simulink model "CNC_3_b"  (R2022b)
settings: Solver=VariableStepAuto  StartTime=0.0  StopTime=0.08  RelTol=1e-3
settings Model: Creator=Mahadevu Sudheer  LastModifiedBy=Mahadevu Sudheer

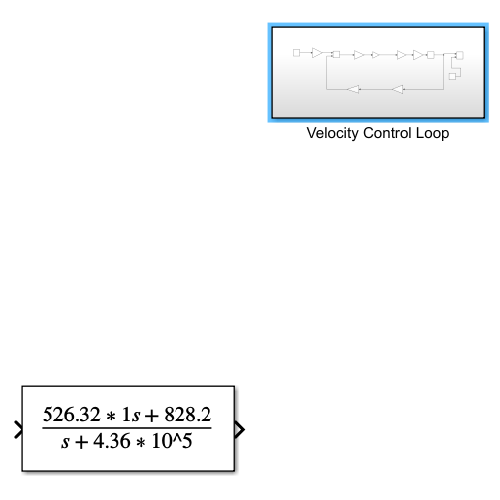
[thumbnail: Simulink's stored preview of the top-level diagram]
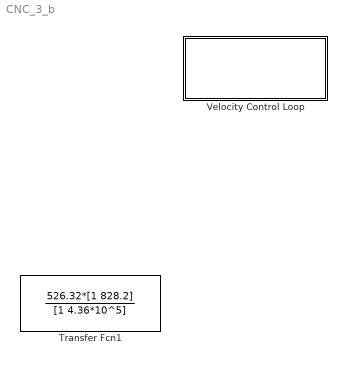
== system CNC_3_b ==
  Transfer Fcn1 : TransferFcn  Numerator=526.32*[1 828.2]  Denominator=[1 4.36*10^5]
  Velocity Control Loop : Subsystem

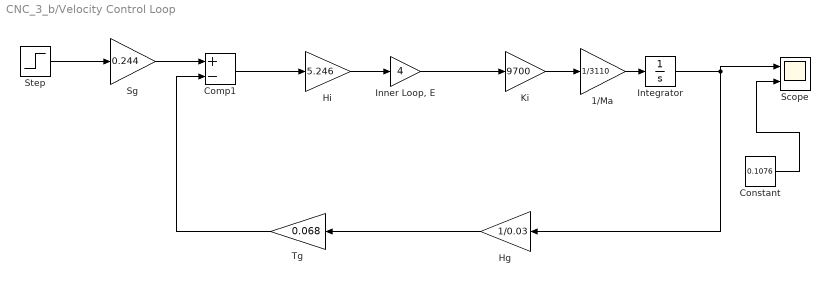
== system CNC_3_b/Velocity Control Loop ==
  1/Ma : Gain  Gain=1/3110
  Comp1 : Sum  Inputs=+-
  Constant : Constant  Value=0.1076
  Hg : Gain  Gain=1/0.03
  Hi : Gain  Gain=5.246
  "Inner Loop, E" : Gain  Gain=4
  Integrator : Integrator
  Ki : Gain  Gain=9700
  Scope : Scope  NumInputPorts=2
  Sg : Gain  Gain=0.244
  Step : Step  Time=0  SampleTime=0
  Tg : Gain  Gain=0.068
  wires:
  Sg/1 -> Comp1/1
  "Inner Loop, E"/1 -> Ki/1
  Ki/1 -> 1/Ma/1
  Hg/1 -> Tg/1
  1/Ma/1 -> Integrator/1
  Integrator/1 -> Scope/1, Hg/1
  Tg/1 -> Comp1/2
  Hi/1 -> "Inner Loop, E"/1
  Comp1/1 -> Hi/1
  Step/1 -> Sg/1
  Constant/1 -> Scope/2
